simulink model "GammaStirlingEngine"  (R2024b)
settings: Solver=ode15s  StartTime=0.0  StopTime=10  RelTol=1e-4  AbsTol=1e-3
PreLoadFcn:
  | GammaStirlingEngineParams;
values from neighbouring files (symbols this model uses):
  ambient = struct()    [GammaStirlingEngineParams.m]
  crank_wheel = struct()    [GammaStirlingEngineParams.m]
  displacer_piston = struct()    [GammaStirlingEngineParams.m]
  flame = struct()    [GammaStirlingEngineParams.m]
  impulse_torque = struct()    [GammaStirlingEngineParams.m]
  power_piston = struct()    [GammaStirlingEngineParams.m]
  regenerator = struct()    [GammaStirlingEngineParams.m]
libraries: fl_lib x45, nesl_utility x11, simulink x1
(part 2 of 2)

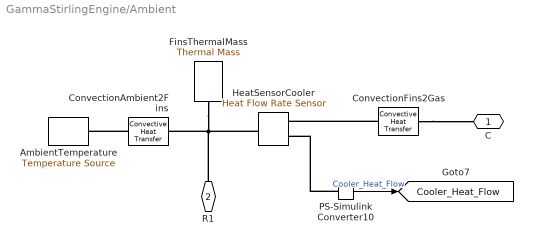
== system GammaStirlingEngine/Ambient ==
  AmbientTemperature : fl_lib/Thermal/Thermal Sources/Temperature Source  temperature=ambient.Temperature K
  ConvectionAmbient2Fins : fl_lib/Thermal/Thermal Elements/Convective Heat Transfer  thermal_type=foundation.enum.constant_variable.constant  area=ambient.ConvAmbient2Fins.area m^2  heat_tr_coeff=ambient.ConvAmbient2Fins.h W/(m^2 * K)  min_heat_tr_coeff=1e-3 W/(K*m^2)  T_specify=off  T_priority=None  T=0 K  T_nominal_specify=off  T_nominal_value=1  T_nominal_unit=K  Q_specify=off  Q_priority=None  Q=0 W  Q_nominal_specify=off  Q_nominal_value=1  Q_nominal_unit=W
  ConvectionFins2Gas : fl_lib/Thermal/Thermal Elements/Convective Heat Transfer  thermal_type=foundation.enum.constant_variable.constant  area=ambient.ConvFins2Gas.area m^2  heat_tr_coeff=ambient.ConvFins2Gas.h W/(m^2 * K)  min_heat_tr_coeff=1e-3 W/(K*m^2)  T_specify=off  T_priority=None  T=0 K  T_nominal_specify=off  T_nominal_value=1  T_nominal_unit=K  Q_specify=off  Q_priority=None  Q=0 W  Q_nominal_specify=off  Q_nominal_value=1  Q_nominal_unit=W
  FinsThermalMass : fl_lib/Thermal/Thermal Elements/Thermal Mass  mass_type=foundation.enum.constant_variable.constant  mass=ambient.Fins.m kg  sp_heat=ambient.Fins.cp J/kg/K  mass_min=1e-6 kg  num_ports=foundation.enum.numPorts2.one  m_specify=off  m_priority=High  m=1 kg  m_nominal_specify=off  m_nominal_value=1  m_nominal_unit=kg  T_specify=on  T_priority=High  T=ambient.Fins.Tinit K  T_nominal_specify=off  T_nominal_value=1  T_nominal_unit=K  Q_specify=off  Q_priority=None  Q=0 W  Q_nominal_specify=off  Q_nominal_value=1  Q_nominal_unit=W
  HeatSensorCooler : fl_lib/Thermal/Thermal Sensors/Heat Flow Rate Sensor
  PS-Simulink Converter10 : nesl_utility/PS-Simulink Converter  PhysicalDomain=network_engine_domain  SubClassName=ps_output  LeftPortType=input  RightPortType=output  PseudoPeriodic=off  Frequencies=[]  VectorFormat=1-D array  Unit=1  AffineConversion=off
  C : PMIOPort  Side=Left
  R1 : PMIOPort  Port=2  Side=Left
  tag scope: Cooler_Heat_Flow=global
  wires:
  PS-Simulink Converter10/1 -> [Cooler_Heat_Flow]  "Cooler_Heat_Flow"
  connections:
  FinsThermalMass/LConn1 -- R1/RConn1 -- HeatSensorCooler/LConn1 -- ConvectionAmbient2Fins/RConn1
  ConvectionAmbient2Fins/LConn1 -- AmbientTemperature/LConn1
  PS-Simulink Converter10/LConn1 -- HeatSensorCooler/RConn1
  ConvectionFins2Gas/LConn1 -- HeatSensorCooler/RConn2
  ConvectionFins2Gas/RConn1 -- C/RConn1

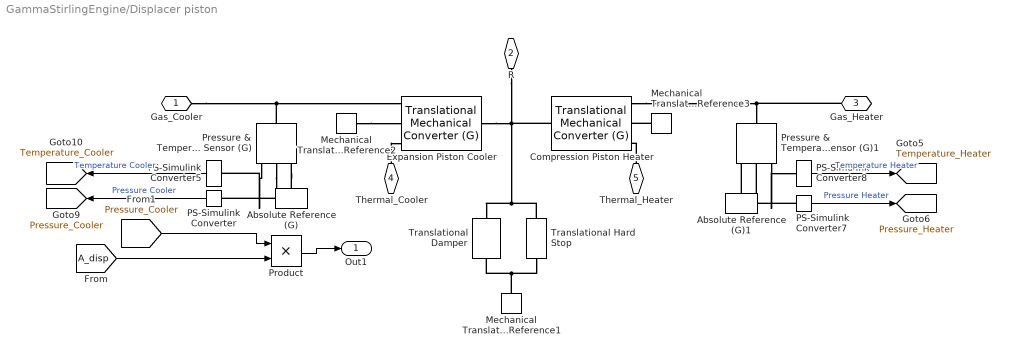
== system GammaStirlingEngine/Displacer piston ==
  Absolute Reference (G) : fl_lib/Gas/Elements/Absolute Reference (G)
      settings: InternalSimscapePortConfiguration="{\"Bottom\":[],\"Left\":[{\"id\":\"A\",\"label\":\"\",\"type\":\"foundation.gas.gas\"}],\"Right\":[],\"Top\":[]}"
  Absolute Reference (G)1 : fl_lib/Gas/Elements/Absolute Reference (G)
      settings: InternalSimscapePortConfiguration="{\"Bottom\":[],\"Left\":[{\"id\":\"A\",\"label\":\"\",\"type\":\"foundation.gas.gas\"}],\"Right\":[],\"Top\":[]}"
  Compression Piston Heater : fl_lib/Gas/Elements/Translational Mechanical Converter (G)  mech_orientation=simscape.enum.posneg.negative  displacement_spec=foundation.enum.DisplacementSpec.Calculate  length_init=displacer_piston.piston.xini_heater m  interface_area=displacer_piston.piston.area_interf m^2  dead_volume=displacer_piston.piston.vol_dead m^3  area_A=displacer_piston.piston.area_A m^2  environment_spec=foundation.enum.pressure_spec.specified  environment_pressure=ambient.pext MPa  p_I_specify=on  p_I_priority=High  p_I=state_init.p0 MPa  p_I_nominal_specify=off  p_I_nominal_value=1  p_I_nominal_unit=MPa  T_I_specify=on  T_I_priority=High  T_I=state_init.T0 K  T_I_nominal_specify=off  T_I_nominal_value=1  T_I_nominal_unit=K  rho_I_specify=off  rho_I_priority=None  rho_I=1.2 kg/m^3  rho_I_nominal_specify=off  rho_I_nominal_value=1  rho_I_nominal_unit=kg/m^3
      settings: InternalSimscapePortConfiguration="{\"Bottom\":[],\"Left\":[{\"id\":\"A\",\"label\":\"A\",\"type\":\"foundation.gas.gas\"},{\"id\":\"C\",\"label\":\"C\",\"type\":\"foundation.mechanical.translational.translational\"},{\"id\":\"H\",\"label\":\"H\",\"type\":\"foundation.thermal.thermal\"}],\"Right\":[{\"id\":\"R\",\"label\":\"R\",\"type\":\"foundation.mechanical.translational.translational\"}],\"Top\":[]}"
  Expansion Piston Cooler : fl_lib/Gas/Elements/Translational Mechanical Converter (G)  mech_orientation=simscape.enum.posneg.positive  displacement_spec=foundation.enum.DisplacementSpec.Calculate  length_init=displacer_piston.piston.xini_cooler m  interface_area=displacer_piston.piston.area_interf m^2  dead_volume=displacer_piston.piston.vol_dead m^3  area_A=displacer_piston.piston.area_A m^2  environment_spec=foundation.enum.pressure_spec.specified  environment_pressure=ambient.pext MPa  p_I_specify=on  p_I_priority=High  p_I=state_init.p0 MPa  p_I_nominal_specify=off  p_I_nominal_value=1  p_I_nominal_unit=MPa  T_I_specify=on  T_I_priority=High  T_I=state_init.T0 K  T_I_nominal_specify=off  T_I_nominal_value=1  T_I_nominal_unit=K  rho_I_specify=off  rho_I_priority=None  rho_I=1.2 kg/m^3  rho_I_nominal_specify=off  rho_I_nominal_value=1  rho_I_nominal_unit=kg/m^3
      settings: InternalSimscapePortConfiguration="{\"Bottom\":[],\"Left\":[{\"id\":\"A\",\"label\":\"A\",\"type\":\"foundation.gas.gas\"},{\"id\":\"C\",\"label\":\"C\",\"type\":\"foundation.mechanical.translational.translational\"},{\"id\":\"H\",\"label\":\"H\",\"type\":\"foundation.thermal.thermal\"}],\"Right\":[{\"id\":\"R\",\"label\":\"R\",\"type\":\"foundation.mechanical.translational.translational\"}],\"Top\":[]}"
  Mechanical Translational Reference1 : fl_lib/Mechanical/Translational Elements/Mechanical Translational Reference
  Mechanical Translational Reference2 : fl_lib/Mechanical/Translational Elements/Mechanical Translational Reference
  Mechanical Translational Reference3 : fl_lib/Mechanical/Translational Elements/Mechanical Translational Reference
  PS-Simulink Converter : nesl_utility/PS-Simulink Converter  PhysicalDomain=network_engine_domain  SubClassName=ps_output  LeftPortType=input  RightPortType=output  PseudoPeriodic=off  Frequencies=[]  VectorFormat=1-D array  Unit=bar  AffineConversion=off
  PS-Simulink Converter5 : nesl_utility/PS-Simulink Converter  PhysicalDomain=network_engine_domain  SubClassName=ps_output  LeftPortType=input  RightPortType=output  PseudoPeriodic=off  Frequencies=[]  VectorFormat=1-D array  Unit=K  AffineConversion=off
  PS-Simulink Converter7 : nesl_utility/PS-Simulink Converter  PhysicalDomain=network_engine_domain  SubClassName=ps_output  LeftPortType=input  RightPortType=output  PseudoPeriodic=off  Frequencies=[]  VectorFormat=1-D array  Unit=bar  AffineConversion=off
  PS-Simulink Converter8 : nesl_utility/PS-Simulink Converter  PhysicalDomain=network_engine_domain  SubClassName=ps_output  LeftPortType=input  RightPortType=output  PseudoPeriodic=off  Frequencies=[]  VectorFormat=1-D array  Unit=K  AffineConversion=off
  Pressure & Temperature Sensor (G) : fl_lib/Gas/Sensors/Pressure & Temperature Sensor (G)  reference=foundation.enum.MeasurementReference.difference  pressure=true  pressure_spec=foundation.enum.PressureMeasementSpec.Absolute  temperature=true
      settings: InternalSimscapePortConfiguration="{\"Bottom\":[{\"id\":\"T\",\"label\":\"T\",\"type\":\"output\"}],\"Left\":[{\"id\":\"A\",\"label\":\"A\",\"type\":\"foundation.gas.gas\"}],\"Right\":[{\"id\":\"B\",\"label\":\"B\",\"type\":\"foundation.gas.gas\"},{\"id\":\"P\",\"label\":\"P\",\"type\":\"output\"}],\"Top\":[]}"
  Pressure & Temperature Sensor (G)1 : fl_lib/Gas/Sensors/Pressure & Temperature Sensor (G)  reference=foundation.enum.MeasurementReference.difference  pressure=true  pressure_spec=foundation.enum.PressureMeasementSpec.Absolute  temperature=true
      settings: InternalSimscapePortConfiguration="{\"Bottom\":[{\"id\":\"T\",\"label\":\"T\",\"type\":\"output\"}],\"Left\":[{\"id\":\"A\",\"label\":\"A\",\"type\":\"foundation.gas.gas\"}],\"Right\":[{\"id\":\"B\",\"label\":\"B\",\"type\":\"foundation.gas.gas\"},{\"id\":\"P\",\"label\":\"P\",\"type\":\"output\"}],\"Top\":[]}"
  Product : Product
  Translational Damper : fl_lib/Mechanical/Translational Elements/Translational Damper  D=displacer_piston.trans_damp N/(m/s)  v_specify=off  v_priority=None  v=0 m/s  v_nominal_specify=off  v_nominal_value=1  v_nominal_unit=m/s  f_specify=off  f_priority=None  f=0 N  f_nominal_specify=off  f_nominal_value=1  f_nominal_unit=N
  Translational Hard Stop : fl_lib/Mechanical/Translational Elements/Translational Hard Stop  upper_bnd=displacer_piston.hardstop.upbound m  lower_bnd=displacer_piston.hardstop.lowbound m  model=simscape.enum.hardstop.smooth  stiff_up=1e7 N/m  stiff_low=1e7 N/m  D_up=1e3 N/(m/s)  D_low=1e3 N/(m/s)  transition=displacer_piston.hardstop.trans_region mm  coeff_rest=0.7  v_tol=0.001 m/s  f_tol=0.001 N  v_specify=off  v_priority=None  v=0 m/s  v_nominal_specify=off  v_nominal_value=1  v_nominal_unit=m/s  f_specify=off  f_priority=None  f=0 N  f_nominal_specify=off  f_nominal_value=1  f_nominal_unit=N  x_specify=on  x_priority=High  x=max(displacer_piston.piston.xini_heater, displacer_piston.piston.xini_cooler) m  x_nominal_specify=off  x_nominal_value=1  x_nominal_unit=m  M_specify=off  M_priority=None  M=0
  Gas_Cooler : PMIOPort  Side=Left
  R : PMIOPort  Port=2  Side=Left
  Gas_Heater : PMIOPort  Port=3  Side=Right
  Thermal_Cooler : PMIOPort  Port=4  Side=Left
  Thermal_Heater : PMIOPort  Port=5  Side=Right
  Out1 : Outport
  tag scope: Pressure_Cooler=global, Pressure_Heater=global, Temperature_Cooler=global, Temperature_Heater=global
  wires:
  PS-Simulink Converter7/1 -> [Pressure_Heater]  "Pressure Heater"
  PS-Simulink Converter8/1 -> [Temperature_Heater]  "Temperature Heater"
  PS-Simulink Converter5/1 -> [Temperature_Cooler]  "Temperature Cooler"
  PS-Simulink Converter/1 -> [Pressure_Cooler]  "Pressure Cooler"
  Product/1 -> Out1/1
  [A_disp] -> Product/2
  [Pressure_Cooler] -> Product/1
  connections:
  Gas_Heater/RConn1 -- Pressure & Temperature Sensor (G)1/LConn1 -- Compression Piston Heater/LConn1
  Mechanical Translational Reference1/LConn1 -- Translational Hard Stop/LConn1 -- Translational Damper/RConn1
  Absolute Reference (G)1/LConn1 -- Pressure & Temperature Sensor (G)1/RConn1
  Pressure & Temperature Sensor (G)/RConn2 -- PS-Simulink Converter/LConn1
  Thermal_Heater/RConn1 -- Compression Piston Heater/LConn3
  Thermal_Cooler/RConn1 -- Expansion Piston Cooler/LConn3
  PS-Simulink Converter7/LConn1 -- Pressure & Temperature Sensor (G)1/RConn2
  Pressure & Temperature Sensor (G)1/RConn3 -- PS-Simulink Converter8/LConn1
  Pressure & Temperature Sensor (G)/RConn3 -- PS-Simulink Converter5/LConn1
  Mechanical Translational Reference3/LConn1 -- Compression Piston Heater/LConn2
  Mechanical Translational Reference2/LConn1 -- Expansion Piston Cooler/LConn2
  Gas_Cooler/RConn1 -- Pressure & Temperature Sensor (G)/LConn1 -- Expansion Piston Cooler/LConn1
  Absolute Reference (G)/LConn1 -- Pressure & Temperature Sensor (G)/RConn1
  Compression Piston Heater/RConn1 -- Expansion Piston Cooler/RConn1 -- Translational Damper/LConn1 -- Translational Hard Stop/RConn1 -- R/RConn1

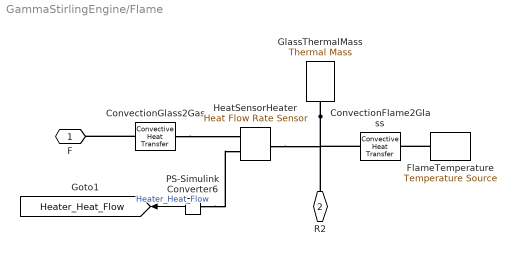
== system GammaStirlingEngine/Flame ==
  ConvectionFlame2Glass : fl_lib/Thermal/Thermal Elements/Convective Heat Transfer  thermal_type=foundation.enum.constant_variable.constant  area=flame.ConvFlame2Glass.area m^2  heat_tr_coeff=flame.ConvFlame2Glass.h W/(m^2 * K)  min_heat_tr_coeff=1e-3 W/(K*m^2)  T_specify=off  T_priority=None  T=0 K  T_nominal_specify=off  T_nominal_value=1  T_nominal_unit=K  Q_specify=off  Q_priority=None  Q=0 W  Q_nominal_specify=off  Q_nominal_value=1  Q_nominal_unit=W
  ConvectionGlass2Gas : fl_lib/Thermal/Thermal Elements/Convective Heat Transfer  thermal_type=foundation.enum.constant_variable.constant  area=flame.ConvGlass2Gas.area m^2  heat_tr_coeff=flame.ConvGlass2Gas.h W/(m^2 * K)  min_heat_tr_coeff=1e-3 W/(K*m^2)  T_specify=off  T_priority=None  T=0 K  T_nominal_specify=off  T_nominal_value=1  T_nominal_unit=K  Q_specify=off  Q_priority=None  Q=0 W  Q_nominal_specify=off  Q_nominal_value=1  Q_nominal_unit=W
  FlameTemperature : fl_lib/Thermal/Thermal Sources/Temperature Source  temperature=flame.Temperature K
  GlassThermalMass : fl_lib/Thermal/Thermal Elements/Thermal Mass  mass_type=foundation.enum.constant_variable.constant  mass=flame.Glass.m kg  sp_heat=flame.Glass.cp J/kg/K  mass_min=1e-6 kg  num_ports=foundation.enum.numPorts2.one  m_specify=off  m_priority=High  m=1 kg  m_nominal_specify=off  m_nominal_value=1  m_nominal_unit=kg  T_specify=on  T_priority=High  T=flame.Glass.Tinit K  T_nominal_specify=off  T_nominal_value=1  T_nominal_unit=K  Q_specify=off  Q_priority=None  Q=0 W  Q_nominal_specify=off  Q_nominal_value=1  Q_nominal_unit=W
  HeatSensorHeater : fl_lib/Thermal/Thermal Sensors/Heat Flow Rate Sensor
  PS-Simulink Converter6 : nesl_utility/PS-Simulink Converter  PhysicalDomain=network_engine_domain  SubClassName=ps_output  LeftPortType=input  RightPortType=output  PseudoPeriodic=off  Frequencies=[]  VectorFormat=1-D array  Unit=1  AffineConversion=off
  F : PMIOPort  Side=Left
  R2 : PMIOPort  Port=2  Side=Left
  tag scope: Heater_Heat_Flow=global
  wires:
  PS-Simulink Converter6/1 -> [Heater_Heat_Flow]  "Heater_Heat_Flow"
  connections:
  GlassThermalMass/LConn1 -- R2/RConn1 -- ConvectionFlame2Glass/RConn1 -- HeatSensorHeater/LConn1
  FlameTemperature/LConn1 -- ConvectionFlame2Glass/LConn1
  PS-Simulink Converter6/LConn1 -- HeatSensorHeater/RConn1
  ConvectionGlass2Gas/RConn1 -- F/RConn1
  ConvectionGlass2Gas/LConn1 -- HeatSensorHeater/RConn2

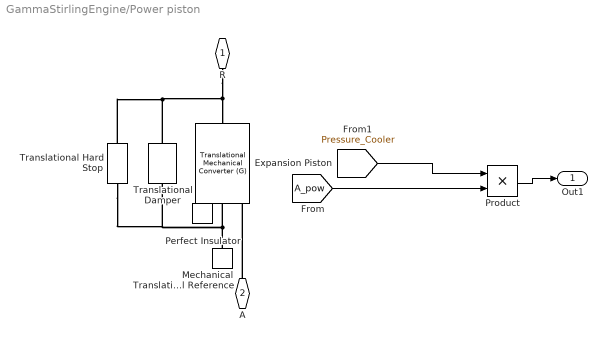
== system GammaStirlingEngine/Power piston ==
  Expansion Piston : fl_lib/Gas/Elements/Translational Mechanical Converter (G)  mech_orientation=simscape.enum.posneg.negative  displacement_spec=foundation.enum.DisplacementSpec.Calculate  length_init=power_piston.piston.xini m  interface_area=power_piston.piston.area_interf m^2  dead_volume=power_piston.piston.vol_dead m^3  area_A=power_piston.piston.area_A m^2  environment_spec=foundation.enum.pressure_spec.specified  environment_pressure=ambient.pext MPa  p_I_specify=on  p_I_priority=High  p_I=state_init.p0 MPa  p_I_nominal_specify=off  p_I_nominal_value=1  p_I_nominal_unit=MPa  T_I_specify=on  T_I_priority=High  T_I=state_init.T0 K  T_I_nominal_specify=off  T_I_nominal_value=1  T_I_nominal_unit=K  rho_I_specify=off  rho_I_priority=Low  rho_I=1.2 kg/m^3  rho_I_nominal_specify=off  rho_I_nominal_value=1  rho_I_nominal_unit=kg/m^3
      settings: InternalSimscapePortConfiguration="{\"Bottom\":[],\"Left\":[{\"id\":\"A\",\"label\":\"A\",\"type\":\"foundation.gas.gas\"},{\"id\":\"C\",\"label\":\"C\",\"type\":\"foundation.mechanical.translational.translational\"},{\"id\":\"H\",\"label\":\"H\",\"type\":\"foundation.thermal.thermal\"}],\"Right\":[{\"id\":\"R\",\"label\":\"R\",\"type\":\"foundation.mechanical.translational.translational\"}],\"Top\":[]}"
  Mechanical Translational Reference : fl_lib/Mechanical/Translational Elements/Mechanical Translational Reference
  Perfect Insulator : fl_lib/Thermal/Thermal Elements/Perfect Insulator  T_specify=off  T_priority=None  T=0 K  T_nominal_specify=off  T_nominal_value=1  T_nominal_unit=K
  Product : Product
  Translational Damper : fl_lib/Mechanical/Translational Elements/Translational Damper  D=power_piston.trans_damp N/(m/s)  v_specify=off  v_priority=None  v=0 m/s  v_nominal_specify=off  v_nominal_value=1  v_nominal_unit=m/s  f_specify=off  f_priority=None  f=0 N  f_nominal_specify=off  f_nominal_value=1  f_nominal_unit=N
  Translational Hard Stop : fl_lib/Mechanical/Translational Elements/Translational Hard Stop  upper_bnd=power_piston.hardstop.upbound m  lower_bnd=power_piston.hardstop.lowbound m  model=simscape.enum.hardstop.smooth  stiff_up=1e7 N/m  stiff_low=1e7 N/m  D_up=1e3 N/(m/s)  D_low=1e3 N/(m/s)  transition=power_piston.hardstop.trans_region mm  coeff_rest=0.7  v_tol=0.001 m/s  f_tol=0.001 N  v_specify=off  v_priority=None  v=0 m/s  v_nominal_specify=off  v_nominal_value=1  v_nominal_unit=m/s  f_specify=off  f_priority=None  f=0 N  f_nominal_specify=off  f_nominal_value=1  f_nominal_unit=N  x_specify=on  x_priority=High  x=power_piston.piston.xini m  x_nominal_specify=off  x_nominal_value=1  x_nominal_unit=m  M_specify=off  M_priority=None  M=0
  R : PMIOPort  Side=Left
  A : PMIOPort  Port=2  Side=Right
  Out1 : Outport
  wires:
  [A_pow] -> Product/2
  [Pressure_Cooler] -> Product/1
  Product/1 -> Out1/1
  connections:
  Mechanical Translational Reference/LConn1 -- Translational Damper/RConn1 -- Translational Hard Stop/LConn1 -- Expansion Piston/LConn2
  Perfect Insulator/LConn1 -- Expansion Piston/LConn3
  A/RConn1 -- Expansion Piston/LConn1
  Translational Hard Stop/RConn1 -- Translational Damper/LConn1 -- R/RConn1 -- Expansion Piston/RConn1

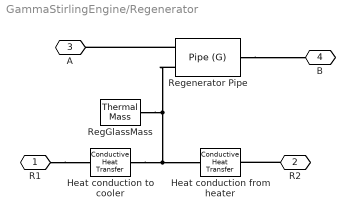
== system GammaStirlingEngine/Regenerator ==
  Heat conduction from heater : fl_lib/Thermal/Thermal Elements/Conductive Heat Transfer  thermal_type=foundation.enum.ConstantVariableTabulated.Constant  wall_geometry=foundation.enum.ConductionWallGeometry.Planar  area=regenerator.conductionHeater.area m^2  thickness=regenerator.conductionHeater.thick m  d_in=0.05 m  d_out=0.1 m  L=1 m  th_cond_min=10 W/(K*m)  th_cond=regenerator.conductionHeater.k W/(m*K)  th_cond_TLU=[413, 401, 392, 383, 371, 357, 342] W/(K*m)  temp_TLU=[200, 273, 400, 600, 800, 1000, 1200] K  T_specify=off  T_priority=None  T=0 K  T_nominal_specify=off  T_nominal_value=1  T_nominal_unit=K  Q_specify=off  Q_priority=None  Q=0 W  Q_nominal_specify=off  Q_nominal_value=1  Q_nominal_unit=W
  Heat conduction to cooler : fl_lib/Thermal/Thermal Elements/Conductive Heat Transfer  thermal_type=foundation.enum.ConstantVariableTabulated.Constant  wall_geometry=foundation.enum.ConductionWallGeometry.Planar  area=regenerator.conductionCooler.area m^2  thickness=regenerator.conductionCooler.thick m  d_in=0.05 m  d_out=0.1 m  L=1 m  th_cond_min=10 W/(K*m)  th_cond=regenerator.conductionCooler.k W/(m*K)  th_cond_TLU=[413, 401, 392, 383, 371, 357, 342] W/(K*m)  temp_TLU=[200, 273, 400, 600, 800, 1000, 1200] K  T_specify=off  T_priority=None  T=0 K  T_nominal_specify=off  T_nominal_value=1  T_nominal_unit=K  Q_specify=off  Q_priority=None  Q=0 W  Q_nominal_specify=off  Q_nominal_value=1  Q_nominal_unit=W
  RegGlassMass : fl_lib/Thermal/Thermal Elements/Thermal Mass  mass_type=foundation.enum.constant_variable.constant  mass=regenerator.mass kg  sp_heat=flame.Glass.cp J/kg/K  mass_min=1e-6 kg  num_ports=foundation.enum.numPorts2.one  m_specify=off  m_priority=High  m=1 kg  m_nominal_specify=off  m_nominal_value=1  m_nominal_unit=kg  T_specify=on  T_priority=High  T=regenerator.initial_temperature K  T_nominal_specify=off  T_nominal_value=1  T_nominal_unit=K  Q_specify=off  Q_priority=None  Q=0 W  Q_nominal_specify=off  Q_nominal_value=1  Q_nominal_unit=W
  Regenerator Pipe : fl_lib/Gas/Elements/Pipe (G)  length=regenerator.geometry.length m  area=regenerator.geometry.area m^2  Dh=regenerator.geometry.hydraulic_diam m  length_add=regenerator.fric_therm.length_add m  roughness=regenerator.fric_therm.roughness m  Re_lam=regenerator.fric_therm.Re_lam  Re_tur=regenerator.fric_therm.Re_tur  shape_factor=regenerator.fric_therm.shape_factor  Nu_lam=regenerator.fric_therm.Nu_lam  p_I_specify=on  p_I_priority=High  p_I=state_init.p0 MPa  p_I_nominal_specify=off  p_I_nominal_value=1  p_I_nominal_unit=MPa  T_I_specify=on  T_I_priority=High  T_I=state_init.T0 K  T_I_nominal_specify=off  T_I_nominal_value=1  T_I_nominal_unit=K  rho_I_specify=off  rho_I_priority=None  rho_I=1.2 kg/m^3  rho_I_nominal_specify=off  rho_I_nominal_value=1  rho_I_nominal_unit=kg/m^3
  R1 : PMIOPort  Side=Left
  R2 : PMIOPort  Port=2  Side=Right
  A : PMIOPort  Port=3  Side=Left
  B : PMIOPort  Port=4  Side=Right
  connections:
  Regenerator Pipe/RConn1 -- B/RConn1
  Regenerator Pipe/LConn1 -- A/RConn1
  Regenerator Pipe/LConn2 -- RegGlassMass/LConn1 -- Heat conduction from heater/RConn1 -- Heat conduction to cooler/LConn1
  R1/RConn1 -- Heat conduction to cooler/RConn1
  R2/RConn1 -- Heat conduction from heater/LConn1

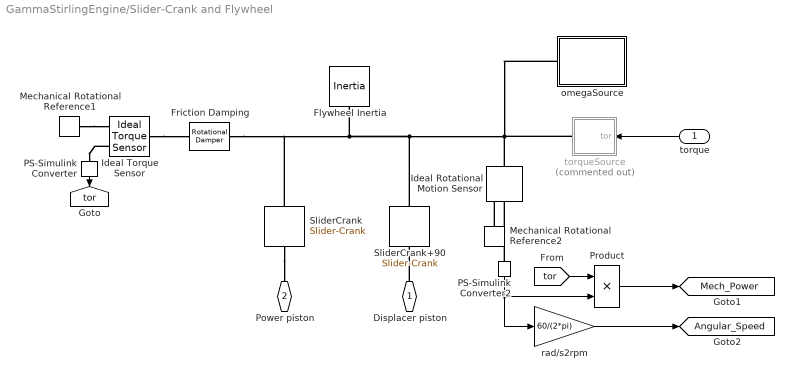
== system GammaStirlingEngine/Slider-Crank and Flywheel ==
  torque : Inport
  Flywheel Inertia : fl_lib/Mechanical/Rotational Elements/Inertia  inertia=crank_wheel.wheel_inertia kg*m^2  num_ports=foundation.enum.numPorts2.one  w_specify=on  w_priority=High  w=0 rad/s  w_nominal_specify=off  w_nominal_value=1  w_nominal_unit=rad/s  t_specify=off  t_priority=None  t=0 N*m  t_nominal_specify=off  t_nominal_value=1  t_nominal_unit=N*m
  Friction Damping : fl_lib/Mechanical/Rotational Elements/Rotational Damper  D=crank_wheel.rot_damp N*m/(rad/s)  w_specify=off  w_priority=None  w=0 rad/s  w_nominal_specify=off  w_nominal_value=1  w_nominal_unit=rad/s  t_specify=off  t_priority=None  t=0 N*m  t_nominal_specify=off  t_nominal_value=1  t_nominal_unit=N*m
  Ideal Rotational Motion Sensor : fl_lib/Mechanical/Mechanical Sensors/Ideal Rotational Motion Sensor  reference=foundation.enum.MeasurementReference.difference  acceleration_port=false  velocity_port=true  position_port=true  wrap_angle=simscape.enum.onoff.off  offset=0 rad
  Ideal Torque Sensor : fl_lib/Mechanical/Mechanical Sensors/Ideal Torque Sensor
  Mechanical Rotational Reference1 : fl_lib/Mechanical/Rotational Elements/Mechanical Rotational Reference
  Mechanical Rotational Reference2 : fl_lib/Mechanical/Rotational Elements/Mechanical Rotational Reference
  PS-Simulink Converter : nesl_utility/PS-Simulink Converter  PhysicalDomain=network_engine_domain  SubClassName=ps_output  LeftPortType=input  RightPortType=output  PseudoPeriodic=off  Frequencies=[]  VectorFormat=1-D array  Unit=N*m  AffineConversion=off
  PS-Simulink Converter2 : nesl_utility/PS-Simulink Converter  PhysicalDomain=network_engine_domain  SubClassName=ps_output  LeftPortType=input  RightPortType=output  PseudoPeriodic=off  Frequencies=[]  VectorFormat=1-D array  Unit=rad/s  AffineConversion=off
  Product : Product
  SliderCrank : fl_lib/Mechanical/Mechanisms/Slider-Crank  crank=crank_wheel.slidercrank_pow.crank_radius m  rod=crank_wheel.slidercrank_pow.rod_length m  inertia=eps kg*m^2  k=1e7 N/m  b=1e3 N/(m/s)  theta_specify=on  theta_priority=High  theta=0 rad  theta_nominal_specify=off  theta_nominal_value=1  theta_nominal_unit=rad  w_specify=off  w_priority=High  w=0 rad/s  w_nominal_specify=off  w_nominal_value=1  w_nominal_unit=rad/s
      settings: InternalSimscapePortConfiguration="{\"Bottom\":[],\"Left\":[{\"id\":\"C\",\"label\":\"C\",\"type\":\"foundation.mechanical.rotational.rotational\"}],\"Right\":[{\"id\":\"S\",\"label\":\"S\",\"type\":\"foundation.mechanical.translational.translational\"}],\"Top\":[]}"
  SliderCrank+90 : fl_lib/Mechanical/Mechanisms/Slider-Crank  crank=crank_wheel.slidercrank_disp.crank_radius m  rod=crank_wheel.slidercrank_disp.rod_length m  inertia=eps kg*m^2  k=1e7 N/m  b=1e3 N/(m/s)  theta_specify=on  theta_priority=High  theta=pi/2 rad  theta_nominal_specify=off  theta_nominal_value=1  theta_nominal_unit=rad  w_specify=on  w_priority=High  w=0 rad/s  w_nominal_specify=off  w_nominal_value=1  w_nominal_unit=rad/s
      settings: InternalSimscapePortConfiguration="{\"Bottom\":[],\"Left\":[{\"id\":\"C\",\"label\":\"C\",\"type\":\"foundation.mechanical.rotational.rotational\"}],\"Right\":[{\"id\":\"S\",\"label\":\"S\",\"type\":\"foundation.mechanical.translational.translational\"}],\"Top\":[]}"
  omegaSource : Subsystem
  rad/s2rpm : Gain  Gain=60/(2*pi)
  torqueSource : Subsystem  Commented=on
  Displacer piston : PMIOPort  Side=Right
  Power piston : PMIOPort  Port=2  Side=Left
  tag scope: Angular_Speed=global, Mech_Power=global, tor=global
  wires:
  PS-Simulink Converter2/1 -> rad/s2rpm/1, Product/2
  [tor] -> Product/1
  Product/1 -> [Mech_Power]
  PS-Simulink Converter/1 -> [tor]
  rad/s2rpm/1 -> [Angular_Speed]
  torque/1 -> torqueSource/1(tor)
  connections:
  Ideal Rotational Motion Sensor/LConn1 -- omegaSource/LConn1 -- torqueSource/RConn1 -- Friction Damping/LConn1 -- SliderCrank/LConn1 -- Flywheel Inertia/LConn1 -- SliderCrank+90/LConn1
  PS-Simulink Converter2/LConn1 -- Ideal Rotational Motion Sensor/RConn2
  Displacer piston/RConn1 -- SliderCrank+90/RConn1
  SliderCrank/RConn1 -- Power piston/RConn1
  Mechanical Rotational Reference2/LConn1 -- Ideal Rotational Motion Sensor/RConn1
  Ideal Torque Sensor/RConn2 -- PS-Simulink Converter/LConn1
  Mechanical Rotational Reference1/LConn1 -- Ideal Torque Sensor/RConn1
  Ideal Torque Sensor/LConn1 -- Friction Damping/RConn1

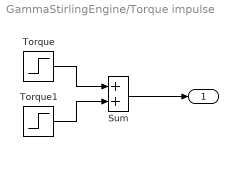
== system GammaStirlingEngine/Torque impulse ==
  Sum : Sum
  Torque : Step  Time=impulse_torque.t_end  Before=impulse_torque.torque  After=0  SampleTime=0
  Torque1 : Step  Time=impulse_torque.t_start  Before=- impulse_torque.torque  After=0  SampleTime=0
  " " : Outport  VectorParamsAs1DForOutWhenUnconnected=off
  wires:
  Torque/1 -> Sum/1
  Torque1/1 -> Sum/2
  Sum/1 -> " "/1

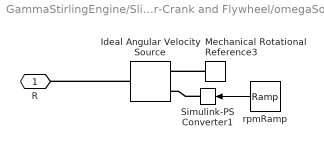
== system GammaStirlingEngine/Slider-Crank and Flywheel/omegaSource ==
  Ideal Angular Velocity Source : fl_lib/Mechanical/Mechanical Sources/Ideal Angular Velocity Source
  Mechanical Rotational Reference3 : fl_lib/Mechanical/Rotational Elements/Mechanical Rotational Reference
  Simulink-PS Converter1 : nesl_utility/Simulink-PS Converter  PhysicalDomain=network_engine_domain  SubClassName=ps_input  LeftPortType=input  RightPortType=output  PseudoPeriodic=off  Frequencies=[]  NoiseDistribution=none  NoiseParameters=[]  Unit=rpm  AffineConversion=off  FilteringAndDerivatives=filter  SimscapeFilterOrder=1  InputFilterTimeConstant=0.001  UdotUserProvided=0
  rpmRamp : simulink/Sources/Ramp  slope=2500/10  start=5  InitialOutput=0
  R : PMIOPort  Side=Left
  wires:
  rpmRamp/1 -> Simulink-PS Converter1/1
  connections:
  Mechanical Rotational Reference3/LConn1 -- Ideal Angular Velocity Source/RConn2
  Simulink-PS Converter1/RConn1 -- Ideal Angular Velocity Source/RConn1
  Ideal Angular Velocity Source/LConn1 -- R/RConn1

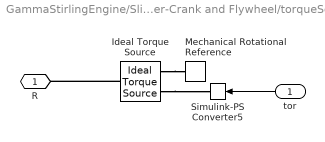
== system GammaStirlingEngine/Slider-Crank and Flywheel/torqueSource ==
  tor : Inport
  Ideal Torque Source : fl_lib/Mechanical/Mechanical Sources/Ideal Torque Source
  Mechanical Rotational Reference : fl_lib/Mechanical/Rotational Elements/Mechanical Rotational Reference
  Simulink-PS Converter5 : nesl_utility/Simulink-PS Converter  PhysicalDomain=network_engine_domain  SubClassName=ps_input  LeftPortType=input  RightPortType=output  PseudoPeriodic=off  Frequencies=[]  NoiseDistribution=none  NoiseParameters=[]  Unit=N*m  AffineConversion=off  FilteringAndDerivatives=provide  SimscapeFilterOrder=1  InputFilterTimeConstant=0.001  UdotUserProvided=0
  R : PMIOPort  Side=Right
  wires:
  tor/1 -> Simulink-PS Converter5/1
  connections:
  Ideal Torque Source/RConn1 -- Simulink-PS Converter5/RConn1
  Ideal Torque Source/RConn2 -- Mechanical Rotational Reference/LConn1
  Ideal Torque Source/LConn1 -- R/RConn1
